simulink model "Simple_test_model_1_2"  (Simulink 8.4)
settings: Solver=FixedStepDiscrete  StartTime=0.0  StopTime="                                                                                 300"  FixedStep=1/256  RelTol=1e-3
undefined symbols (not defined in the file): currentCFG_one_sub_model_UB, UB
libraries: gRTanalyze x3, Tools x1, gUSBamplib x1
settings Model: Creator=2110973l  LastModifiedBy=2110973l
settings DataIOCC: SignalLoggingSaveFormat=Dataset
settings OptimizationCC: ExpressionDepthLimit=128
settings DebuggingCC: UnderspecifiedInitializationDetection=Simplified  MergeDetectMultiDrivingBlocksExec=error  FcnCallInpInsideContextMsg=EnableAllAsError  StateNameClashWarn=none
settings GRTTargetCC: CombineOutputUpdateFcns=on  GRTInterface=off

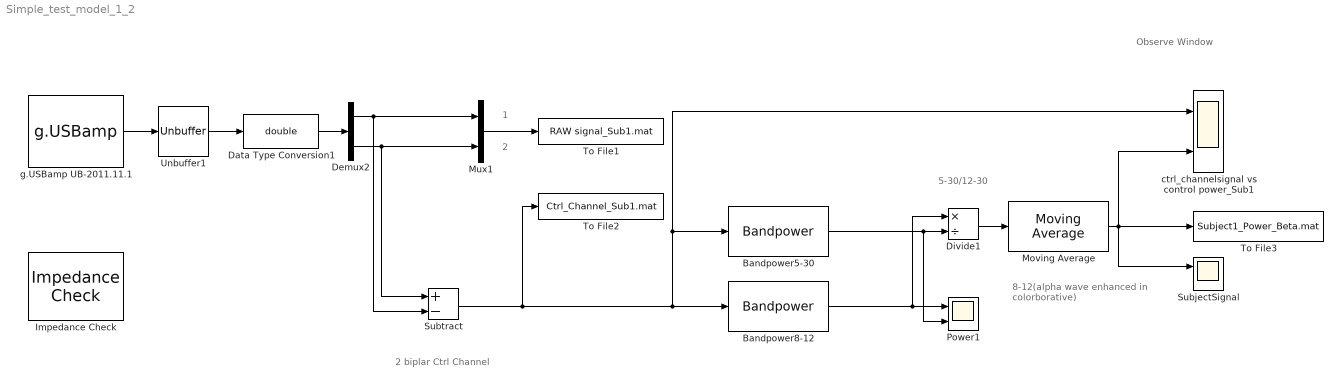
== system Simple_test_model_1_2 ==
  note: 2
  note: 1
  note: Observe Window
  note: 2 biplar Ctrl Channel
  note: 8-12(alpha wave enhanced in colorborative)
  note: 5-30/12-30
  Bandpower5-30 : gRTanalyze/Bandpower  Order=5  LowerFreq=5  UpperFreq=30  WindowLength=128
  Bandpower8-12 : gRTanalyze/Bandpower  Order=5  LowerFreq=8  UpperFreq=12  WindowLength=128
  Data Type Conversion1 : DataTypeConversion  OutDataTypeStr=double
  Demux2 : Demux  Outputs=2
  Divide1 : Product  Inputs=*/
  Impedance Check : Tools/Impedance Check  SystemSampleTime=-1
  Moving Average : gRTanalyze/Moving Average  windowSize=256
  Mux1 : Mux  Inputs=2
  Power1 : Scope  NumInputPorts=2
      settings: YMin=0~0  YMax=1200~1200  SaveName=ScopeData4
  SubjectSignal : Scope  NumInputPorts=2
      settings: YMin=1.014~-1  YMax=1.032~1  SaveName=ScopeData8
  Subtract : Sum  Inputs=+-
  To File1 : ToFile  Filename=RAW signal_Sub1.mat  MatrixName=AllChannel
  To File2 : ToFile  Filename=Ctrl_Channel_Sub1.mat  MatrixName=Ctrl_Channel
  To File3 : ToFile  Filename=Subject1_Power_Beta.mat  MatrixName=Subject1_Power_Beta
  Unbuffer1 : Unbuffer  SampleBasedProcessing=Same as frame based
  ctrl_channelsignal vs control power_Sub1 : Scope  NumInputPorts=2
      settings: YMin=-100~0  YMax=100~20  SaveName=ScopeData9
  g.USBamp UB-2011.11.1 : gUSBamplib/g.USBamp  cfg=currentCFG_one_sub_model_UB-2011.11.31.cfg  snr=UB-2011.11.31
  wires:
  Bandpower8-12/1 -> Divide1/1, Power1/1
  Bandpower5-30/1 -> Divide1/2, Power1/2
  Moving Average/1 -> To File3/1, ctrl_channelsignal vs control power_Sub1/2, SubjectSignal/1
  Divide1/1 -> Moving Average/1
  g.USBamp UB-2011.11.1/1 -> Unbuffer1/1
  Unbuffer1/1 -> Data Type Conversion1/1
  Data Type Conversion1/1 -> Demux2/1
  Demux2/1 -> Subtract/2, Mux1/1
  Subtract/1 -> Bandpower5-30/1, ctrl_channelsignal vs control power_Sub1/1, Bandpower8-12/1, To File2/1
  Demux2/2 -> Subtract/1, Mux1/2
  Mux1/1 -> To File1/1
